simulink model "WS2Sol"  (R2019b)
settings: Solver=VariableStepAuto  StartTime=0.0  StopTime=20  RelTol=1e-3
libraries: simulink_extras x6
settings Model: Creator=Shishir  LastModifiedBy=Shishir

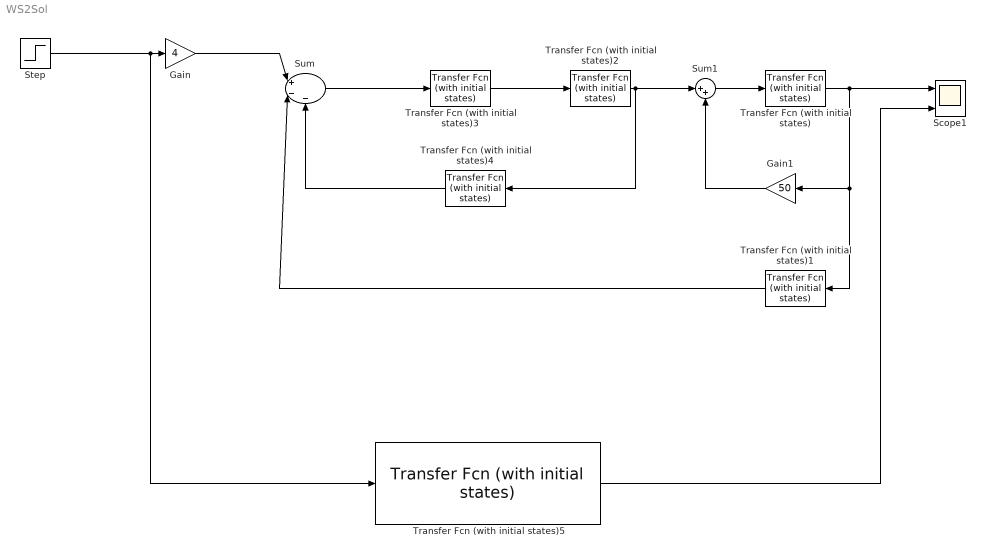
== system WS2Sol ==
  Gain : Gain  Gain=4
  Gain1 : Gain  Gain=50
  Scope1 : Scope  NumInputPorts=2
  Step : Step  Time=0  SampleTime=0
  Sum : Sum  Inputs=|+--
  Sum1 : Sum  Inputs=|++
  Transfer Fcn (with initial states) : simulink_extras/Additional Linear/Transfer Fcn (with initial states)  N=[1]  D="[1  0 0]"  X0=0
  Transfer Fcn (with initial states)1 : simulink_extras/Additional Linear/Transfer Fcn (with initial states)  N=[1 0 2]  D=[1 0 0 14]  X0=0
  Transfer Fcn (with initial states)2 : simulink_extras/Additional Linear/Transfer Fcn (with initial states)  N=[1 0]  D="[1  0 2]"  X0=0
  Transfer Fcn (with initial states)3 : simulink_extras/Additional Linear/Transfer Fcn (with initial states)  N=[1]  D="[1  1]"  X0=0
  Transfer Fcn (with initial states)4 : simulink_extras/Additional Linear/Transfer Fcn (with initial states)  N=[4 2]  D="[1  2 1]"  X0=0
  Transfer Fcn (with initial states)5 : simulink_extras/Additional Linear/Transfer Fcn (with initial states)  N=[4 8 4 56 112 56 0]  D=[1 3 -45 -125 -200 -1177 -2344 -3485 -7668 -5598 -1400]  X0=0
  wires:
  Step/1 -> Transfer Fcn (with initial states)5/1, Gain/1
  Gain/1 -> Sum/1
  Sum/1 -> Transfer Fcn (with initial states)3/1
  Transfer Fcn (with initial states)3/1 -> Transfer Fcn (with initial states)2/1
  Transfer Fcn (with initial states)2/1 -> Transfer Fcn (with initial states)4/1, Sum1/1
  Sum1/1 -> Transfer Fcn (with initial states)/1
  Gain1/1 -> Sum1/2
  Transfer Fcn (with initial states)/1 -> Transfer Fcn (with initial states)1/1, Gain1/1, Scope1/1
  Transfer Fcn (with initial states)1/1 -> Sum/2
  Transfer Fcn (with initial states)4/1 -> Sum/3
  Transfer Fcn (with initial states)5/1 -> Scope1/2
